simulink model "w2pr3"  (R2020b)
settings: Solver=VariableStepAuto  StartTime=0.0  StopTime=10.0  RelTol=1e-3
model workspace (MAT data in the model file):
  Ki = 40
  Kp = 1500
  b = 50
  m = 1000
settings Model: Creator=user  LastModifiedBy=user

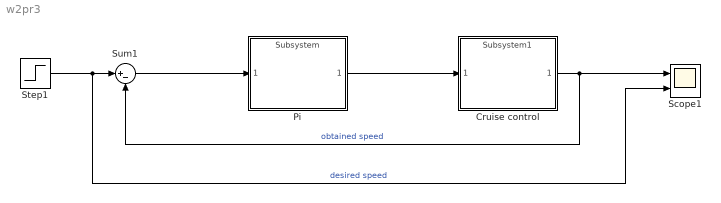
== system w2pr3 ==
  Cruise control : ModelReference  ModelNameDialog=Subsystem1  SimulationMode=Normal  ModelReferenceVersion=1.2
  Pi : ModelReference  ModelNameDialog=Subsystem  SimulationMode=Normal  ModelReferenceVersion=1.2
  Scope1 : Scope  NumInputPorts=2
  Step1 : Step  SampleTime=0
  Sum1 : Sum  Inputs=|+-
  wires:
  Pi/1 -> Cruise control/1
  Sum1/1 -> Pi/1
  Cruise control/1 -> Scope1/1, Sum1/2  "obtained speed"
  Step1/1 -> Scope1/2, Sum1/1  "desired speed"
